simulink model "CVF"  (R2018a)
settings: Solver=FixedStepAuto  StartTime=0.0  StopTime=2  FixedStep=0.0001  RelTol=1e-3
values from neighbouring files (symbols this model uses):
  Tm = 0.1/5    (= 0.02)    [Init.m]
libraries: simulink x3, powerlib_meascontrol x3
settings Model: Creator=Augusto  LastModifiedBy=Augusto

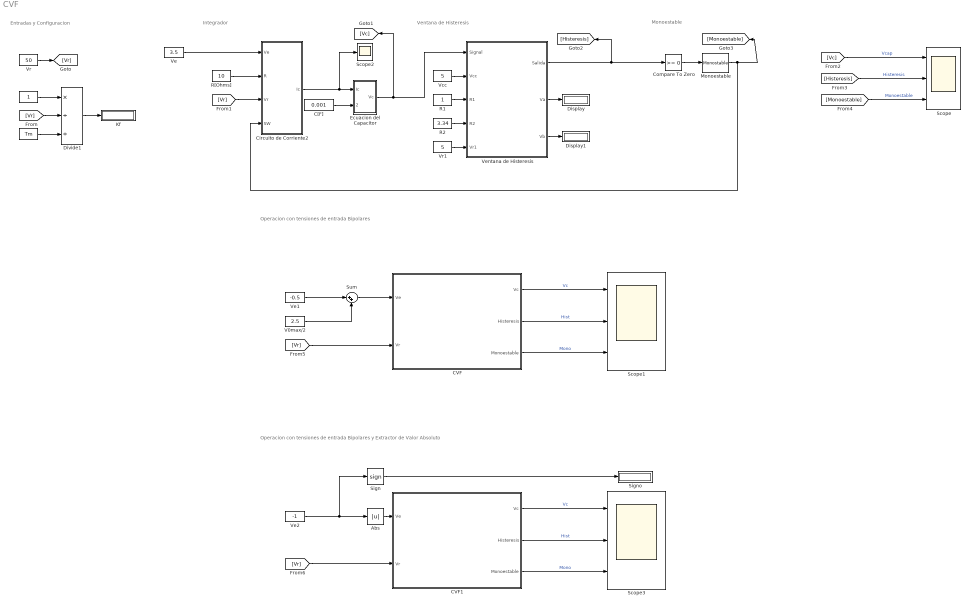
== system CVF ==
  note: Operacion con tensiones de entrada Bipolares
  note: Monoestable
  note: Ventana de Histeresis
  note: Integrador
  note: Entradas y Configuracion
  note: Operacion con tensiones de entrada Bipolares y Extractor de Valor Absoluto
  " " : Constant  Value=Tm
  "   " : Constant
  Abs : Abs
  CVF : Subsystem
  CVF1 : Subsystem
  C[F] : Constant  Value=0.001
  Circuito de Corriente2 : Subsystem
  Compare To Zero : simulink/Logic and Bit Operations/Compare To Zero  relop=>=  OutDataTypeStr=boolean
  Display : Display
  Display1 : Display
  Divide1 : Product  Inputs=*//
  Ecuacion del Capacitor : Subsystem
  Kf : Display
  "Monoestable " : powerlib_meascontrol/Logic/Monostable  EdgeDetect=Falling  PulseDuration=Tm  ic=1  Ts=0
      settings: SourceProductName=Simscape Power Systems  SourceProductBaseCode=PS
  R1 : Constant
  R2 : Constant  Value=3.34
  "R[Ohms] " : Constant  Value=10
  Scope : Scope  NumInputPorts=3
  Scope1 : Scope  NumInputPorts=3
  Scope2 : Scope
  Scope3 : Scope  NumInputPorts=3
  Sign : Signum
  Signo : Display
  Sum : Sum  Inputs=|++
  V0max/2 : Constant  Value=2.5
  Vcc : Constant  Value=5
  Ve : Constant  Value=3.5
  Ve1 : Constant  Value=-0.5
  Ve2 : Constant  Value=-1
  Ventana de Histeresis : MATLAB Function  TreatAsAtomicUnit=on
  Vr : Constant  Value=50
  Vr1 : Constant  Value=5
  wires:
  Ve/1 -> Circuito de Corriente2/1(Ve)
  "R[Ohms] "/1 -> Circuito de Corriente2/2(R)
  Circuito de Corriente2/1(Ic) -> Scope2/1, Ecuacion del Capacitor/1(Ic)
  C[F]/1 -> Ecuacion del Capacitor/2(Cap)
  Vcc/1 -> Ventana de Histeresis/2(Vcc)
  R1/1 -> Ventana de Histeresis/3(R1)
  R2/1 -> Ventana de Histeresis/4(R2)
  Vr1/1 -> Ventana de Histeresis/5(Vr1)
  Ventana de Histeresis/1(Salida) -> Compare To Zero/1, [Histeresis]
  Vr/1 -> [Vr]
  [Vr] -> Divide1/2
  [Vr] -> Circuito de Corriente2/3(Vr)
  " "/1 -> Divide1/3
  "   "/1 -> Divide1/1
  Divide1/1 -> Kf/1
  [Vc] -> Scope/1  "Vcap"
  [Histeresis] -> Scope/2  "Histeresis"
  Ventana de Histeresis/2(Va) -> Display/1
  Ventana de Histeresis/3(Vb) -> Display1/1
  Compare To Zero/1 -> "Monoestable "/1
  [Monoestable] -> Scope/3  "Monoestable"
  Ecuacion del Capacitor/1(Vc) -> [Vc], Ventana de Histeresis/1(Signal)
  "Monoestable "/1 -> Circuito de Corriente2/4(SW), [Monoestable]
  Sum/1 -> CVF/1(Ve)
  Ve1/1 -> Sum/1
  V0max/2/1 -> Sum/2
  CVF/3(Monoestable) -> Scope1/3  "Mono"
  [Vr] -> CVF/2(Vr)
  CVF/1(Vc) -> Scope1/1  "Vc"
  CVF/2(Histeresis) -> Scope1/2  "Hist"
  CVF1/2(Histeresis) -> Scope3/2  "Hist"
  [Vr] -> CVF1/2(Vr)
  Ve2/1 -> Sign/1, Abs/1
  CVF1/3(Monoestable) -> Scope3/3  "Mono"
  CVF1/1(Vc) -> Scope3/1  "Vc"
  Abs/1 -> CVF1/1(Ve)
  Sign/1 -> Signo/1

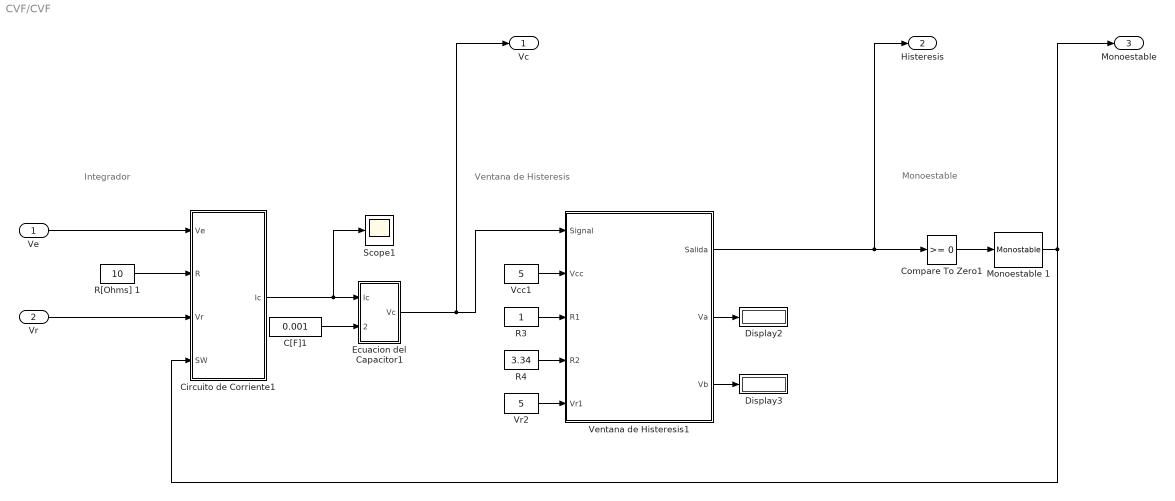
== system CVF/CVF ==
  note: Ventana de Histeresis
  note: Monoestable
  note: Integrador
  Ve : Inport
  Vr : Inport  Port=2
  C[F]1 : Constant  Value=0.001
  Circuito de Corriente1 : Subsystem
  Compare To Zero1 : simulink/Logic and Bit Operations/Compare To Zero  relop=>=  OutDataTypeStr=boolean
  Display2 : Display
  Display3 : Display
  Ecuacion del Capacitor1 : Subsystem
  Monoestable 1 : powerlib_meascontrol/Logic/Monostable  EdgeDetect=Falling  PulseDuration=Tm  ic=1  Ts=0
      settings: SourceProductName=Simscape Power Systems  SourceProductBaseCode=PS
  R3 : Constant
  R4 : Constant  Value=3.34
  R[Ohms] 1 : Constant  Value=10
  Scope1 : Scope
  Vcc1 : Constant  Value=5
  Ventana de Histeresis1 : MATLAB Function  TreatAsAtomicUnit=on
  Vr2 : Constant  Value=5
  Vc : Outport
  Histeresis : Outport  Port=2
  Monoestable : Outport  Port=3
  wires:
  Vcc1/1 -> Ventana de Histeresis1/2(Vcc)
  Ventana de Histeresis1/3(Vb) -> Display3/1
  Ventana de Histeresis1/2(Va) -> Display2/1
  Ventana de Histeresis1/1(Salida) -> Histeresis/1, Compare To Zero1/1
  R[Ohms] 1/1 -> Circuito de Corriente1/2(R)
  Ecuacion del Capacitor1/1(Vc) -> Vc/1, Ventana de Histeresis1/1(Signal)
  Vr2/1 -> Ventana de Histeresis1/5(Vr1)
  Compare To Zero1/1 -> Monoestable 1/1
  Circuito de Corriente1/1(Ic) -> Scope1/1, Ecuacion del Capacitor1/1(Ic)
  R3/1 -> Ventana de Histeresis1/3(R1)
  C[F]1/1 -> Ecuacion del Capacitor1/2(Cap)
  R4/1 -> Ventana de Histeresis1/4(R2)
  Vr/1 -> Circuito de Corriente1/3(Vr)
  Monoestable 1/1 -> Monoestable/1, Circuito de Corriente1/4(SW)
  Ve/1 -> Circuito de Corriente1/1(Ve)

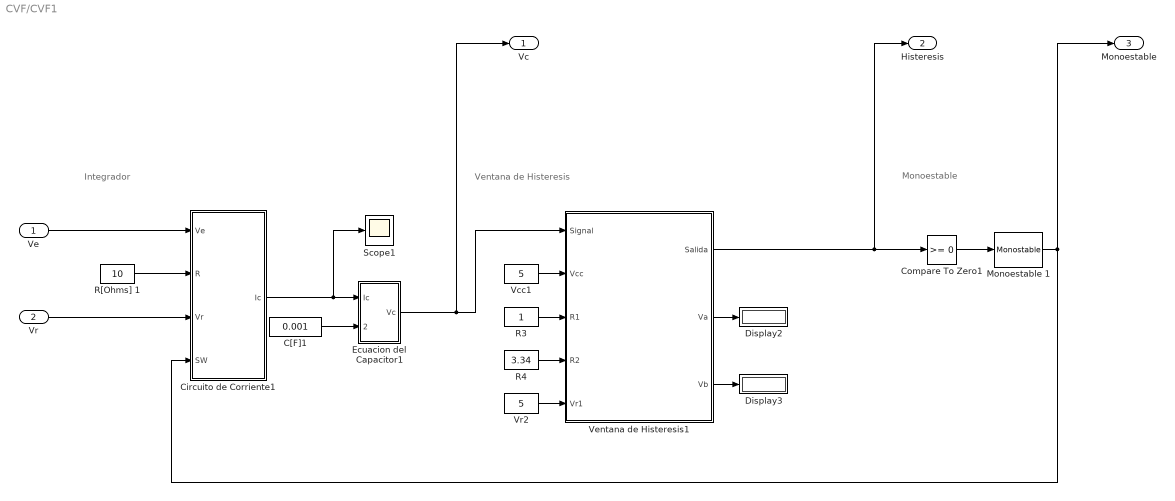
== system CVF/CVF1 ==
  note: Ventana de Histeresis
  note: Monoestable
  note: Integrador
  Ve : Inport
  Vr : Inport  Port=2
  C[F]1 : Constant  Value=0.001
  Circuito de Corriente1 : Subsystem
  Compare To Zero1 : simulink/Logic and Bit Operations/Compare To Zero  relop=>=  OutDataTypeStr=boolean
  Display2 : Display
  Display3 : Display
  Ecuacion del Capacitor1 : Subsystem
  Monoestable 1 : powerlib_meascontrol/Logic/Monostable  EdgeDetect=Falling  PulseDuration=Tm  ic=1  Ts=0
      settings: SourceProductName=Simscape Power Systems  SourceProductBaseCode=PS
  R3 : Constant
  R4 : Constant  Value=3.34
  R[Ohms] 1 : Constant  Value=10
  Scope1 : Scope
  Vcc1 : Constant  Value=5
  Ventana de Histeresis1 : MATLAB Function  TreatAsAtomicUnit=on
  Vr2 : Constant  Value=5
  Vc : Outport
  Histeresis : Outport  Port=2
  Monoestable : Outport  Port=3
  wires:
  Vcc1/1 -> Ventana de Histeresis1/2(Vcc)
  Ventana de Histeresis1/3(Vb) -> Display3/1
  Ventana de Histeresis1/2(Va) -> Display2/1
  Ventana de Histeresis1/1(Salida) -> Histeresis/1, Compare To Zero1/1
  R[Ohms] 1/1 -> Circuito de Corriente1/2(R)
  Ecuacion del Capacitor1/1(Vc) -> Vc/1, Ventana de Histeresis1/1(Signal)
  Vr2/1 -> Ventana de Histeresis1/5(Vr1)
  Compare To Zero1/1 -> Monoestable 1/1
  Circuito de Corriente1/1(Ic) -> Scope1/1, Ecuacion del Capacitor1/1(Ic)
  R3/1 -> Ventana de Histeresis1/3(R1)
  C[F]1/1 -> Ecuacion del Capacitor1/2(Cap)
  R4/1 -> Ventana de Histeresis1/4(R2)
  Vr/1 -> Circuito de Corriente1/3(Vr)
  Monoestable 1/1 -> Monoestable/1, Circuito de Corriente1/4(SW)
  Ve/1 -> Circuito de Corriente1/1(Ve)

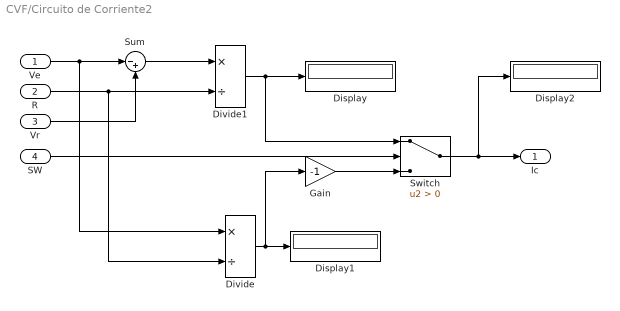
== system CVF/Circuito de Corriente2 ==
  Ve : Inport
  R : Inport  Port=2
  Vr : Inport  Port=3
  SW : Inport  Port=4
  Display : Display
  Display1 : Display
  Display2 : Display
  Divide : Product  Inputs=*/
  Divide1 : Product  Inputs=*/
  Gain : Gain  Gain=-1
  Sum : Sum  Inputs=|-+
  Switch : Switch  Criteria=u2 > Threshold
  Ic : Outport
  wires:
  Ve/1 -> Divide/1, Sum/1
  SW/1 -> Switch/2
  Sum/1 -> Divide1/1
  Divide/1 -> Display1/1, Gain/1
  Divide1/1 -> Display/1, Switch/1
  Vr/1 -> Sum/2
  R/1 -> Divide/2, Divide1/2
  Switch/1 -> Display2/1, Ic/1
  Gain/1 -> Switch/3

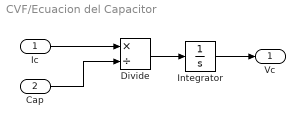
== system CVF/Ecuacion del Capacitor ==
  Ic : Inport
  Cap : Inport  Port=2
  Divide : Product  Inputs=*/
  Integrator : Integrator
  Vc : Outport
  wires:
  Ic/1 -> Divide/1
  Integrator/1 -> Vc/1
  Divide/1 -> Integrator/1
  Cap/1 -> Divide/2

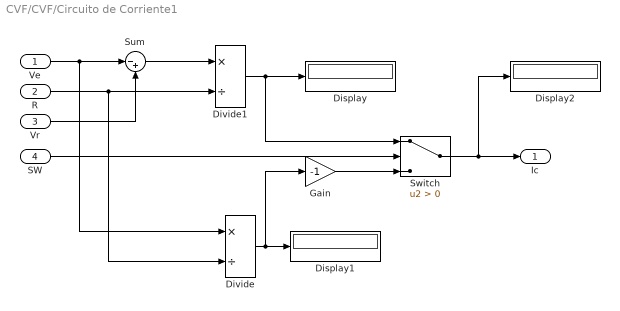
== system CVF/CVF/Circuito de Corriente1 ==
  Ve : Inport
  R : Inport  Port=2
  Vr : Inport  Port=3
  SW : Inport  Port=4
  Display : Display
  Display1 : Display
  Display2 : Display
  Divide : Product  Inputs=*/
  Divide1 : Product  Inputs=*/
  Gain : Gain  Gain=-1
  Sum : Sum  Inputs=|-+
  Switch : Switch  Criteria=u2 > Threshold
  Ic : Outport
  wires:
  Ve/1 -> Divide/1, Sum/1
  SW/1 -> Switch/2
  Sum/1 -> Divide1/1
  Divide/1 -> Display1/1, Gain/1
  Divide1/1 -> Display/1, Switch/1
  Vr/1 -> Sum/2
  R/1 -> Divide/2, Divide1/2
  Switch/1 -> Display2/1, Ic/1
  Gain/1 -> Switch/3

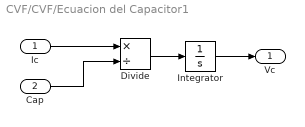
== system CVF/CVF/Ecuacion del Capacitor1 ==
  Ic : Inport
  Cap : Inport  Port=2
  Divide : Product  Inputs=*/
  Integrator : Integrator
  Vc : Outport
  wires:
  Ic/1 -> Divide/1
  Integrator/1 -> Vc/1
  Divide/1 -> Integrator/1
  Cap/1 -> Divide/2

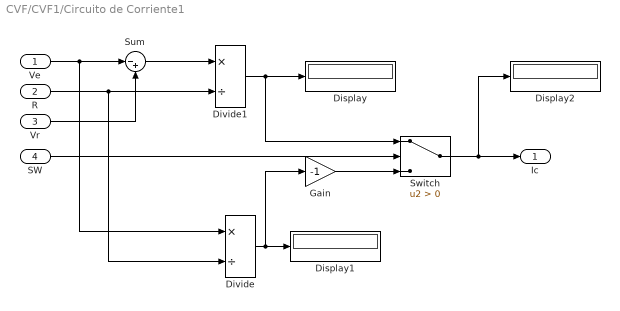
== system CVF/CVF1/Circuito de Corriente1 ==
  Ve : Inport
  R : Inport  Port=2
  Vr : Inport  Port=3
  SW : Inport  Port=4
  Display : Display
  Display1 : Display
  Display2 : Display
  Divide : Product  Inputs=*/
  Divide1 : Product  Inputs=*/
  Gain : Gain  Gain=-1
  Sum : Sum  Inputs=|-+
  Switch : Switch  Criteria=u2 > Threshold
  Ic : Outport
  wires:
  Ve/1 -> Divide/1, Sum/1
  SW/1 -> Switch/2
  Sum/1 -> Divide1/1
  Divide/1 -> Display1/1, Gain/1
  Divide1/1 -> Display/1, Switch/1
  Vr/1 -> Sum/2
  R/1 -> Divide/2, Divide1/2
  Switch/1 -> Display2/1, Ic/1
  Gain/1 -> Switch/3

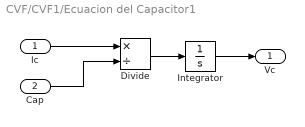
== system CVF/CVF1/Ecuacion del Capacitor1 ==
  Ic : Inport
  Cap : Inport  Port=2
  Divide : Product  Inputs=*/
  Integrator : Integrator
  Vc : Outport
  wires:
  Ic/1 -> Divide/1
  Integrator/1 -> Vc/1
  Divide/1 -> Integrator/1
  Cap/1 -> Divide/2

== matlab function CVF/Ventana de Histeresis1 ==
  settings: updateMethod=DISCRETE
  data: Signal input; Salida output; Vcc input; R1 input; R2 input; Vr1 input; Va output; Vb output
function [Salida,Va,Vb]= fcn(Signal,Vcc,R1,R2,Vr1)
     
    persistent u 
    if isempty(u)
        u=Vcc;
        Va = 0;
        Vb = 0;
    
    else
        epsilon = Vcc*(R1/R2);
        VR1 = -Vr1*(R1+R2)/R2;
        Va = VR1 - epsilon;
        Vb = VR1 + epsilon;
        if(Signal<=Va) 
            u = -Vcc;
        end
        if(Signal>=Vb)
            u = Vcc;
        end
    end
    
    Salida = u;

== matlab function CVF/Ventana de Histeresis ==
  settings: updateMethod=DISCRETE
  data: Signal input; Salida output; Vcc input; R1 input; R2 input; Vr1 input; Va output; Vb output
function [Salida,Va,Vb]= fcn(Signal,Vcc,R1,R2,Vr1)
     
    persistent u 
    if isempty(u)
        u=Vcc;
        Va = 0;
        Vb = 0;
    
    else
        epsilon = Vcc*(R1/R2);
        VR1 = -Vr1*(R1+R2)/R2;
        Va = VR1 - epsilon;
        Vb = VR1 + epsilon;
        if(Signal<=Va) 
            u = -Vcc;
        end
        if(Signal>=Vb)
            u = Vcc;
        end
    end
    
    Salida = u;

== matlab function CVF/CVF1/Ventana de Histeresis1 ==
  settings: updateMethod=DISCRETE
  data: Signal input; Salida output; Vcc input; R1 input; R2 input; Vr1 input; Va output; Vb output
function [Salida,Va,Vb]= fcn(Signal,Vcc,R1,R2,Vr1)
     
    persistent u 
    if isempty(u)
        u=Vcc;
        Va = 0;
        Vb = 0;
    
    else
        epsilon = Vcc*(R1/R2);
        VR1 = -Vr1*(R1+R2)/R2;
        Va = VR1 - epsilon;
        Vb = VR1 + epsilon;
        if(Signal<=Va) 
            u = -Vcc;
        end
        if(Signal>=Vb)
            u = Vcc;
        end
    end
    
    Salida = u;
